simulink model "motorSim"  (R2017a)
settings: Solver=VariableStepAuto  StartTime=0.0  StopTime=30.0  MaxStep=0.01  RelTol=1e-3
settings Model: Creator=default  LastModifiedBy=default

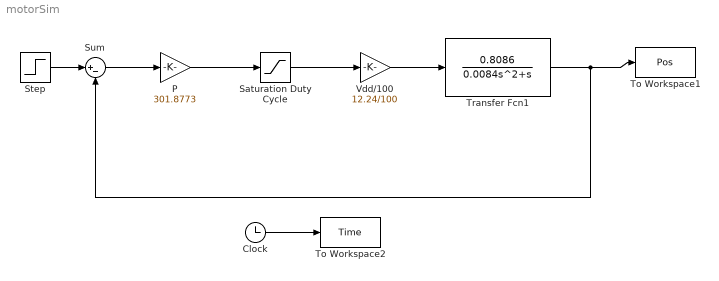
== system motorSim ==
  Clock : Clock
  P : Gain  Gain=301.8773
  Saturation Duty Cycle : Saturate  UpperLimit=100  LowerLimit=0
  Step : Step  Time=0  SampleTime=0
  Sum : Sum  Inputs=|+-
  To Workspace1 : ToWorkspace  VariableName=Pos  SampleTime=-1
  To Workspace2 : ToWorkspace  VariableName=Time  SampleTime=-1
  Transfer Fcn1 : TransferFcn  Numerator=[0.8086]  Denominator=[0.0084 1 0]
  Vdd/100 : Gain  Gain=12.24/100
  wires:
  Sum/1 -> P/1
  Transfer Fcn1/1 -> To Workspace1/1, Sum/2
  Clock/1 -> To Workspace2/1
  Saturation Duty Cycle/1 -> Vdd/100/1
  Vdd/100/1 -> Transfer Fcn1/1
  Step/1 -> Sum/1
  P/1 -> Saturation Duty Cycle/1
